simulink model "dbuildv3p0"  (R2025a)
settings: Solver=FixedStepAuto  StartTime=0.0  StopTime=inf  FixedStep=0.002  RelTol=1e-3
model workspace (MAT data in the model file):
  A_busbar = 0.0015
  A_pack = 0.711626248
  C = 400
  C_nominal = 3
  GR = 13.75
  I_max = 157.708978328
  Izz = 76.97
  P = 5
  P_DD = 1
  REGEN_GAIN = 1
  R_e = 0.197
  S = 138
  SW_TV_GAIN = 0.0250298750679
  SoC_initial = 1
  TC_CUT = 20
  T_amb = 297.15
  Tmax = 21
  W_max = 34
  a = 0.7497
  brakebias = 0.5
  busbar_CC_area = 0.000108
  busbar_Cp = 237
  busbar_length = 0.032
  busbar_mass = 0.01
  busbar_resistivity = 1.68e-08
  busbar_thermalcontact_resistance = 1
  c_factor = 0.244
  cell_Cp = 1000
  cell_mass = 0.046
  deg_to_rad = 0.0174533
  g = 9.81
  h_busbar = 5
  h_pack = 5
  kappa_thresh = 0.12
  l = 1.53
  mpersec_to_kph = 3.6
  rackdisp_to_steerangle = 1.29615626969
  rad_to_deg = 57.2958
  rpm_to_radpers = 0.10472
  trigger_pressure = 4.65396
undefined symbols (not defined in the file or in its folder): TC_switch, TV_switch
libraries: eeGeneralControl x2, Solver_SF x1, sl3dlib x1, simulink x1
(part 2 of 2)

== system dbuildv3p0/DiL Functionality/Brake system/Rear braking system/Proportioning valve ==
  rear master cylinder pressure : Inport
  Product : Product
  proportioning constant LUT : Lookup_n-D  BreakpointsForDimension1=[1.03421;2.48211;3.93001;4.65396;5.37791;6.82581;8.273709]  BreakpointsForDimension2=[2.06843;4.13685;6.20528;8.273709;10.34214]  Table=[0.71666667 0.57333333 0.52555556 0.50166667 0.48733333;1 0.77166667 0.65777778 0.6008333300000001 0.56666667;1 0.97166667 0.79111111 0.70083333 0.64666667;1 1 0.85777778 0.75083333 0.68666667;1 1 0.92444444 0.8 0.72666667;1 1 1 0.9 0.806;1 1 1 1 0.886]  InterpMethod=Akima spline  InternalRulePriority=Speed  RndMeth=Simplest
      settings: InputPortMap=u0,u1
  trigger pressure : Constant  Value=trigger_pressure
  proportioning valve pressure : Outport
  wires:
  trigger pressure/1 -> proportioning constant LUT/1
  rear master cylinder pressure/1 -> Product/2, proportioning constant LUT/2
  Product/1 -> proportioning valve pressure/1
  proportioning constant LUT/1 -> Product/1

== system dbuildv3p0/DiL Functionality/Driver inputs/Button Box/Simulation off ==
  Power button status : Inport
  Stop Simulation : Stop
  wires:
  Power button status/1 -> Stop Simulation/1

== system dbuildv3p0/DiL Functionality/Driver inputs/Button Box/TC control ==
  TC power button : Inport
  Change Detector : eeGeneralControl/Change Detector  VariantControl=Variant1  LabelModeActiveChoice=Discrete  ChangeType=Rising edge  x0=0  Ts=-1
      settings: LibrarySourceBlock=ee_sl_lib/General Control/Change Detector
  If : If  IfExpression=u1 == 1
  If Action Subsystem : Subsystem  TreatAsAtomicUnit=on
  Terminator : Terminator
  TC switch : Outport
  wires:
  TC power button/1 -> Change Detector/1
  If/2 -> Terminator/1
  If/1 -> If Action Subsystem/Action
  If Action Subsystem/1(TC switch) -> TC switch/1
  Change Detector/1 -> If/1

== system dbuildv3p0/DiL Functionality/Driver inputs/Button Box/TV control ==
  TV power button : Inport
  Change Detector : eeGeneralControl/Change Detector  VariantControl=Variant1  LabelModeActiveChoice=Discrete  ChangeType=Rising edge  x0=0  Ts=-1
      settings: LibrarySourceBlock=ee_sl_lib/General Control/Change Detector
  If : If  IfExpression=u1 == 1
  If Action Subsystem : Subsystem  TreatAsAtomicUnit=on
  Terminator : Terminator
  TV switch : Outport
  wires:
  TV power button/1 -> Change Detector/1
  If/2 -> Terminator/1
  If/1 -> If Action Subsystem/Action
  If Action Subsystem/1(TV switch) -> TV switch/1
  Change Detector/1 -> If/1

== system dbuildv3p0/Battery Thermal Model/Battery Cells/Battery Heat Generation/Current Estimator/Power Estimator ==
  Add : Sum
  Gain : Gain  Gain=rpm_to_radpers
  Gain2 : Gain  Gain=rpm_to_radpers
  Product : Product
  Product1 : Product
  Scope : Scope
      settings: ActiveDisplayYMinimum=-386.82091  ActiveDisplayYMaximum=3481.38823
  Motor Power (W) : Outport
  wires:
  [omega_RL] -> Gain/1
  [CMD_RL] -> Product/1
  Gain/1 -> Product/2
  Gain2/1 -> Product1/2
  [CMD_RR] -> Product1/1
  [omega_RR] -> Gain2/1
  Product/1 -> Scope/1, Add/1  "Left Motor Power (W)"
  Product1/1 -> Add/2  "Right Motor Power (W)"
  Add/1 -> Motor Power (W)/1  "Motor Power (W)"

== system dbuildv3p0/Control System/Driver Assists/Torque Vectoring/Target Yaw Rate Estimator/Slip Angle Estimator ==
  note: \arctan\left(\frac{a}{R}\right)
  Front : Subsystem
  Rear : Subsystem

== system dbuildv3p0/Control System/Driver Assists/Torque Vectoring/Target Yaw Rate Estimator/Yaw Rate Error ==
  r_est : Inport
  Mux : Mux  Inputs=2
  Sum : Sum  Inputs=|+-
  To File : ToFile  Filename=yawrate.mat
      settings: Decimation=3
  To File1 : ToFile  Filename=targetyawrate.mat
      settings: Decimation=3
  To File2 : ToFile  Filename=yawrateerror.mat
      settings: Decimation=3
  Yaw Rate Error Scope : Scope
      settings: ActiveDisplayYMinimum=-14.16098  ActiveDisplayYMaximum=13.33266
  Yaw Rate Scope : Scope
      settings: ActiveDisplayYMinimum=-139.01553  ActiveDisplayYMaximum=139.20732  DataLoggingVariableName=ScopeData2
  tag scope: r_error=global
  wires:
  r_est/1 -> Mux/1, Sum/1, To File1/1  "Target Yaw Rate (deg/s)"
  [r] -> Mux/2, To File/1, Sum/2  "Yaw Rate (deg/s)"
  Sum/1 -> To File2/1, [r_error], Yaw Rate Error Scope/1  "Yaw Rate Error (deg/s)"
  Mux/1 -> Yaw Rate Scope/1

== system dbuildv3p0/Control System/Driver Assists/Traction Control/Vx Estimation/Ax to Vx ==
  Ax : Inport
  Omega Vx : Inport  Port=2
  Enable : EnablePort
  Integrator : Integrator
  Plus : Sum
  to m/s^2 : Gain  Gain=g
  Ax Vx : Outport
  wires:
  Ax/1 -> to m/s^2/1
  Integrator/1 -> Plus/2
  Omega Vx/1 -> Plus/1
  Plus/1 -> Ax Vx/1
  to m/s^2/1 -> Integrator/1

== system dbuildv3p0/Control System/Driver Assists/Traction Control/Vx Estimation/Method Enabler ==
  BRK_F : Inport
  Constant : Constant  Value=0
  Constant1 : Constant
  Constant2 : Constant  Value=0
  Constant3 : Constant
  Switch : Switch  Criteria=u2 > Threshold  Threshold=0.1  SaturateOnIntegerOverflow=off  InputSameDT=off
  Switch1 : Switch  Criteria=u2 > Threshold  SaturateOnIntegerOverflow=off  InputSameDT=off
  Enable Ax method : Outport
  Enable omega method : Outport  Port=2
  wires:
  Constant1/1 -> Switch/3
  Constant/1 -> Switch/1
  BRK_F/1 -> Switch/2
  Constant2/1 -> Switch1/1
  Constant3/1 -> Switch1/3
  Switch1/1 -> Enable Ax method/1
  Switch/1 -> Enable omega method/1, Switch1/2

== system dbuildv3p0/Control System/Driver Assists/Traction Control/Vx Estimation/omega to Vx ==
  omega : Inport
  Enable : EnablePort
  Gain : Gain  Gain=R_e
  Gain1 : Gain  Gain=rpm_to_radpers
  Vx : Outport
  wires:
  omega/1 -> Gain1/1
  Gain/1 -> Vx/1
  Gain1/1 -> Gain/1

== system dbuildv3p0/DiL Functionality/Driver inputs/Button Box/TC control/If Action Subsystem ==
  Action Port : ActionPort
  Add : Sum
  Constant1 : Constant  Value=-1
  Constant2 : Constant
  Display : Display
  Memory : Memory  InitialCondition=TC_switch  LinearizeMemory=on
  Switch : Switch  Criteria=u2 > Threshold  SaturateOnIntegerOverflow=off  InputSameDT=off
  TC switch : Outport
  wires:
  Constant2/1 -> Switch/3
  Constant1/1 -> Switch/1
  Memory/1 -> TC switch/1, Display/1, Switch/2, Add/1
  Add/1 -> Memory/1
  Switch/1 -> Add/2

== system dbuildv3p0/DiL Functionality/Driver inputs/Button Box/TV control/If Action Subsystem ==
  Action Port : ActionPort
  Add : Sum
  Constant1 : Constant  Value=-1
  Constant2 : Constant
  Display : Display
  Memory : Memory  InitialCondition=TV_switch  LinearizeMemory=on
  Switch : Switch  Criteria=u2 > Threshold  SaturateOnIntegerOverflow=off  InputSameDT=off
  TV switch : Outport
  wires:
  Constant2/1 -> Switch/3
  Constant1/1 -> Switch/1
  Memory/1 -> TV switch/1, Display/1, Switch/2, Add/1
  Add/1 -> Memory/1
  Switch/1 -> Add/2

== system dbuildv3p0/Control System/Driver Assists/Torque Vectoring/Target Yaw Rate Estimator/Slip Angle Estimator/Front ==
  Atan : Trigonometry  Operator=atan
  Constant : Constant  Value=a
  Divide : Product  Inputs=*/
  Divide1 : Product  Inputs=*/
  Gain : Gain  Gain=c_factor
  Gain1 : Gain  Gain=rackdisp_to_steerangle
  Gain2 : Gain  Gain=1/3.6
  Gain3 : Gain  Gain=g
  Square : Math  Operator=square
  Sum : Sum  Inputs=|+-
  tag scope: alpha_F=global
  wires:
  [delta_SW] -> Gain/1  "Steering Wheel Angle (deg)"
  Gain/1 -> Gain1/1  "Rack Displacement (mm)"
  Gain1/1 -> Sum/2  "Front Wheel Steering Angle (deg)"
  [Vx] -> Gain2/1  "Vehicle Velocity (kph)"
  Gain2/1 -> Square/1  "Vehicle Velocity (m/s)"
  Square/1 -> Divide/1
  [Ay] -> Gain3/1  "Lateral Acceleration (G)"
  Gain3/1 -> Divide/2  "Lateral Acceleration (m/s^2)"
  Divide/1 -> Divide1/2  "Turning Radius (m)"
  Constant/1 -> Divide1/1  "CG to Front Wheel Distance (m)"
  Atan/1 -> Sum/1  "Slip Angle w/o Steering (deg)"
  Divide1/1 -> Atan/1
  Sum/1 -> [alpha_F]  "Front Wheel Slip Angle (deg)"

== system dbuildv3p0/Control System/Driver Assists/Torque Vectoring/Target Yaw Rate Estimator/Slip Angle Estimator/Rear ==
  Atan : Trigonometry  Operator=atan
  Constant : Constant  Value=l-a
  Divide : Product  Inputs=*/
  Divide1 : Product  Inputs=*/
  Gain2 : Gain  Gain=1/3.6
  Gain3 : Gain  Gain=g
  Square : Math  Operator=square
  tag scope: alpha_R=global
  wires:
  Divide/1 -> Divide1/2  "Turning Radius (m)"
  [Ay] -> Gain3/1  "Lateral Acceleration (G)"
  Atan/1 -> [alpha_R]  "Rear Wheel Slip Angle (deg)"
  Gain3/1 -> Divide/2  "Lateral Acceleration (m/s^2)"
  [Vx] -> Gain2/1  "Vehicle Velocity (kph)"
  Square/1 -> Divide/1
  Constant/1 -> Divide1/1  "CG to Rear Wheel Distance (m)"
  Gain2/1 -> Square/1  "Vehicle Velocity (m/s)"
  Divide1/1 -> Atan/1
